simulink model "Plant0"  (R2020b)
settings: Solver=FixedStepDiscrete  StartTime=0.0  StopTime=3  FixedStep=1e-06  RelTol=1e-3  EnableMultiTasking=on
settings Model: ExtModeTrigDuration=2  Creator=拾夕  LastModifiedBy=拾夕
settings DataIOCC: SaveOutput=off  SaveTime=off
settings OptimizationCC: DefaultUnderspecifiedDataType=single  EnhancedBackFolding=on  PassReuseOutputArgsAs=Individual arguments  ZeroExternalMemoryAtStartup=off  ZeroInternalMemoryAtStartup=off  MaxStackSize=64  OptimizeBlockOrder=speed  DifferentSizesBufferReuse=on  OptimizationCustomize=off  EfficientTunableParamExpr=on
settings DebuggingCC: ParameterTunabilityLossMsg=error
settings HardwareCC: ProdBitPerInt=16  ProdBitPerPointer=16  ProdBitPerSizeT=16  ProdBitPerPtrDiffT=16  ProdLargestAtomicFloat=None  ProdWordSize=8  ProdHWDeviceType=Atmel->AVR
settings SFSimCC: MATLABDynamicMemAlloc=off
settings RTWCC: Description=Embedded Coder  SystemTargetFile=ert.tlc  HardwareBoard=Arduino Uno  GenCodeOnly=on  TemplateMakefile=ert_default_tmf  GenerateReport=on  RetainRTWFile=on  Toolchain=Arduino AVR  BuildConfiguration=Faster Runs  LaunchReport=on  GenerateWebview=on  GenerateCodeMetricsReport=on
settings CodeAppCC: ForceParamTrailComments=on  IgnoreCustomStorageClasses=off  OperatorAnnotations=on  SimulinkDataObjDesc=on  SFDataObjDesc=on  InsertBlockDesc=on
settings ERTTargetCC: SupportContinuousTime=on  SupportVariableSizeSignals=on  ExtModeStaticAllocSize=250

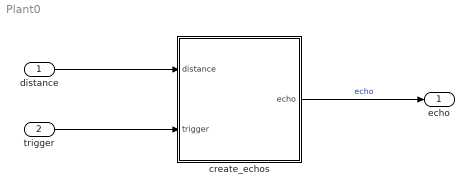
== system Plant0 ==
  distance : Inport  OutDataTypeStr=single  PortDimensions=1
  trigger : Inport  Port=2  OutDataTypeStr=single  PortDimensions=1  SampleTime=[9.9999999999999995e-07,0]
  create_echos : Stateflow chart  TreatAsAtomicUnit=on
  echo : Outport  OutDataTypeStr=single  PortDimensions=1  SampleTime=[9.9999999999999995e-07,0]
  wires:
  trigger/1 -> create_echos/2(trigger)
  create_echos/1(echo) -> echo/1  "echo"
  distance/1 -> create_echos/1(distance)

== stateflow chart Plant0/create_echos ==
  state CreateZero
    en:
    echo=0;
  state CreateOne
    en:
    echo=1;
  (default) -> CreateZero
  CreateZero -> CreateOne : [trigger==1&&distance<=400&&distance>=2]
  CreateOne -> CreateZero : after(distance*58,usec)
  data: distance input single; trigger input single; echo output single
